simulink model "sim_inverter_MA"  (R2022a)
settings: Solver=FixedStepDiscrete  StartTime=0.0  StopTime=5  FixedStep=Ts  RelTol=1e-3
PreLoadFcn:
  | sim_params;
InitFcn:
  | sim_params;
values from neighbouring files (symbols this model uses):
  capacitor_C = 0.00033    [sim_datadict.sldd]
  capacitor_R = 0.03    [sim_datadict.sldd]
  freq_ref = 60.0    [sim_datadict.sldd]
  fsw = 10000    [run_simulation.m]    (also in sim_params.m)
  I_ref = 6.5    [sim_datadict.sldd]
  Ki_i = 36.06    [sim_params.m]
  Ki_vd = Ki    (= 341.85)    [sim_params.m]
  Ki_vq = Ki    (= 341.85)    [sim_params.m]
  Kp_i = 0.0405    [sim_params.m]
  Kp_vd = Kp    (= 3.68799083448)    [sim_params.m]
  Kp_vq = Kp    (= 3.68799083448)    [sim_params.m]
  source_L = {0, 0.3e-3, 0.6e-3, 1e-3, 1.8e-3, 3.5e-3, 5e-3, 8e-3, 15e-3, 25e-3, 165e-3}    [load_sim_space.m]    (also in run_inverterSims.m = {0, 0.3e-3, 0.6e-3, 1e-3, 1.8e-3, 3.5e-3, 5e-3, 8e-3, 15e-3,; sim_datadict.sldd = 0.001)
  source_R = {0, 0.1, 0.2, 0.3, 0.5, 1, 1.5, 2.5, 5, 8, 12.5}    [load_sim_space.m]    (also in run_inverterSims.m = {0, 0.1, 0.2, 0.3, 0.5, 1, 1.5, 2.5, 5, 8}; sim_datadict.sldd = 0.1)
  Ts = 1e-6    (= 1e-06)    [run_simulation.m]    (also in sim_params.m)
  Vref = 380    [load_control_params.m]    (also in sim_params.m)
libraries: slpidlib x3, spsRMSLib x3, spsThreePhaseVIMeasurementLib x2, spsAsynchronousMachineSIUnitsLib x1, spsAlphaBetaZerotoabcLib x1, spsAlphaBetaZerotodq0Lib x1, eeAsmScalarControl x1, eeGeneralControl x1, eePwmGeneratorTwoLevel x1, spsabctoAlphaBetaZeroLib x1, spsdq0toAlphaBetaZeroLib x1, spsThreePhaseSourceLib x1
settings Model: DataDictionary=sim_datadict.sldd  ARTEMISmethode_block_infos=$$__separator__$$  SimulationMode=accelerator  Creator=thale  LastModifiedBy=thale
settings DataIOCC: LimitDataPoints=on  MaxDataPoints=1/Ts  SaveFormat=Array  SaveOutput=off  DSMLogging=off  SaveTime=off  ReturnWorkspaceOutputs=off  TimeSaveName=time  LoggingIntervals=[0, inf]

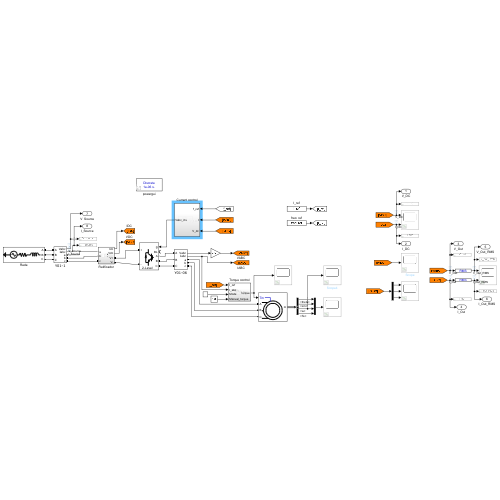
[thumbnail: Simulink's stored preview of the top-level diagram]
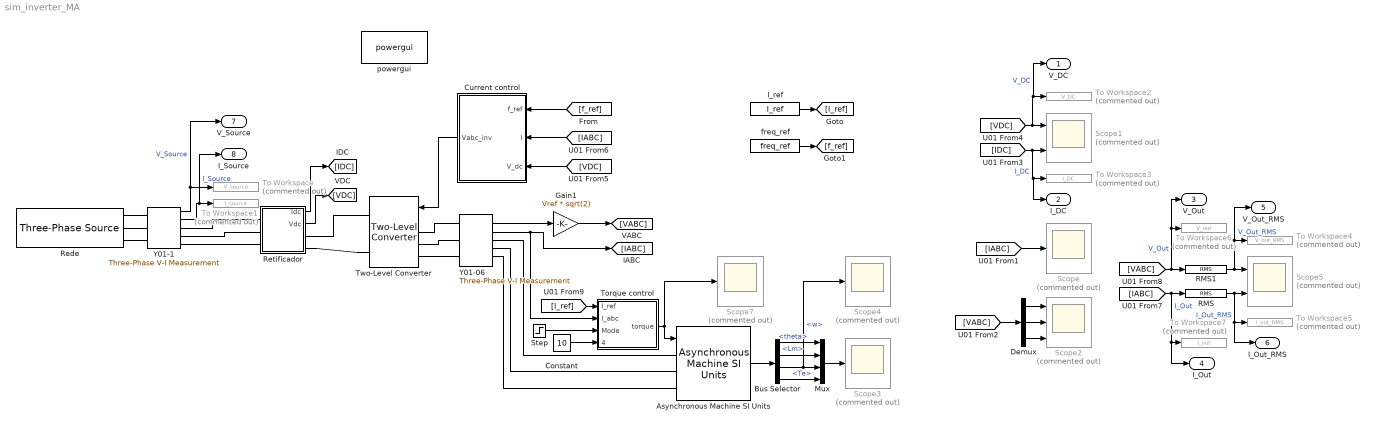
== system sim_inverter_MA ==
  Asynchronous Machine SI Units : spsAsynchronousMachineSIUnitsLib/Asynchronous Machine SI Units  RotorType=Squirrel-cage  PresetModel=No  MechanicalLoad=Torque Tm  ShowDetailedParameters=on  ReferenceFrame=Rotor  Units=SI  MeasurementBus=on  NominalParameters=[3000 380 60]  VoltageRatio=1  Stator=[0.6837 0.004152]  Rotor=[0.451 0.004152]  Cage1=[0.4155 0.002066]  Cage2=[0.4168 0.0003495]  Lm=0.1486  Mechanical=[0.0120 0.008141 2]  PolePairs=2  InitialConditions=[0 0 0 0 0 0 0 0]  SimulateSaturation=off  Saturation=[14.03593122, 27.81365428, 53.79336849, 72.68890987, 97.98006896, 148.6815601, 215.7428561, 302.9841135, 428.7778367 ; 230, 322, 414, 460, 506, 552, 598, 644, 690]  LoadFlowParameters=1492000  TsPowergui=0  TsBlock=-1  IterativeModel=Trapezoidal non iterative  IterativeDiscreteModel=Trapezoidal non iterative  Pmec=1.492e+006
  Bus Selector : BusSelector  OutputSignals=theta,Lm,w,Te
  Constant : Constant  Value=10
  Current control : Subsystem
  Demux : Demux  Outputs=3
  Gain1 : Gain  Gain=Vref * sqrt(2)
  I_ref : Constant  Value=I_ref
  Mux : Mux
  RMS : spsRMSLib/RMS  TrueRMS=off  Freq=freq_ref  RMSInit=0  Ts=Ts
  RMS1 : spsRMSLib/RMS  TrueRMS=off  Freq=freq_ref  RMSInit=0  Ts=Ts
  Rede : spsThreePhaseSourceLib/Three-Phase Source  InternalConnection=Yg  VoltagePhases=off  Voltage=Vref  PhaseAngle=0  Voltage_phases=[25e3 25e3 25e3]/sqrt(3)  PhaseAngles_phases=[0 -120 +120]  Frequency=60  NonIdealSource=on  SpecifyImpedance=off  Resistance=source_R  Inductance=source_L  ShortCircuitLevel=100e6  BaseVoltage=Vref  XRratio=7  BusType=swing  Pref=10e3  Qref=0  Prefabc=[10e3, 10e3, 10e3]  Qrefabc=[0, 0, 0]  Qmin=-inf  Qmax=inf
  Retificador : Subsystem
  Scope{,3..4,7} (4 alike) : Scope  Commented=on
  Scope1 : Scope  Commented=on  NumInputPorts=2
  Scope2 : Scope  Commented=on  NumInputPorts=3
  Scope5 : Scope  Commented=on  NumInputPorts=2
  Step : Step  Time=0.5  SampleTime=0
  To Workspace : ToWorkspace  Commented=on  VariableName=V_source  SampleTime=-1
      settings: MaxDataPoints=1/Ts  Save2DSignal=2-D array (concatenate along first dimension)
  To Workspace1 : ToWorkspace  Commented=on  VariableName=I_source  SampleTime=-1
      settings: Save2DSignal=2-D array (concatenate along first dimension)
  To Workspace2 : ToWorkspace  Commented=on  VariableName=V_DC  SampleTime=-1
      settings: MaxDataPoints=1/Ts  Save2DSignal=2-D array (concatenate along first dimension)
  To Workspace3 : ToWorkspace  Commented=on  VariableName=I_DC  SampleTime=-1
      settings: MaxDataPoints=1/Ts  Save2DSignal=2-D array (concatenate along first dimension)
  To Workspace4 : ToWorkspace  Commented=on  VariableName=V_out_RMS  SampleTime=-1
      settings: MaxDataPoints=1/Ts  Save2DSignal=2-D array (concatenate along first dimension)
  To Workspace5 : ToWorkspace  Commented=on  VariableName=I_out_RMS  SampleTime=-1
      settings: Save2DSignal=2-D array (concatenate along first dimension)
  To Workspace6 : ToWorkspace  Commented=on  VariableName=V_out  SampleTime=-1
      settings: MaxDataPoints=1/Ts  Save2DSignal=2-D array (concatenate along first dimension)
  To Workspace7 : ToWorkspace  Commented=on  VariableName=I_out  SampleTime=-1
      settings: MaxDataPoints=1/Ts  Save2DSignal=2-D array (concatenate along first dimension)
  Torque control : Subsystem
  Two-Level Converter : spsTwoLevelConverterLib/Two-Level Converter  ModelType=Switching devices  Ron=1e-3  Rs=1e6  Cs=inf  Vforward=[0,0]  Ron_Diode=1e-3  Rs_Diode=1e6  Cs_Diode=inf  Vf_Diode=1e-3  Rs_CurrentSource=inf  Ron_ACsource=1e-3
      settings: SourceProductBaseCode=PS
  Y01-06 : spsThreePhaseVIMeasurementLib/Three-Phase V-I Measurement  VoltageMeasurement=phase-to-ground  SetLabelV=off  LabelV=Vabc  Vpu=on  VpuLL=off  CurrentMeasurement=yes  SetLabelI=off  LabelI=Iabc  Ipu=off  Pbase=100e6  Vbase=Vref  OutputType=Complex  PhasorSimulation=off  PSBequivalent=0
  Y01-1 : spsThreePhaseVIMeasurementLib/Three-Phase V-I Measurement  VoltageMeasurement=phase-to-ground  SetLabelV=off  LabelV=Vabc  Vpu=off  VpuLL=off  CurrentMeasurement=yes  SetLabelI=off  LabelI=Iabc  Ipu=off  Pbase=100e6  Vbase=Vref  OutputType=Complex  PhasorSimulation=off  PSBequivalent=0
  freq_ref : Constant  Value=freq_ref
  powergui : spspowerguiLib/powergui  Priority=1  SimulationMode=Discrete  SampleTime=Ts  frequency=60  Iterations=50  frequencyindice=0  Pbase=100e6  ErrMax=1e-4  UnitsV=kV  UnitsW=MW  buscounter=0  FunctionMessages=off  echomessages=off  EnableUseOfTLC=off  CurrentSourceSwitches=off  DisableSnubberDevices=off  DisableRonSwitches=off  DisableVfSwitches=off  DisplayEquations=off  AutomaticDiscreteSolvers=off  SolverType=Tustin/Backward Euler (TBE)  Interpol=off  ExternalGateDelay=off  methode=off  Ts=100  x0status=blocks  SPID=on  SwTol=0  HookPort=off  NonlinearTolerance=1e-4  nMaxIteration=100  ContinueOnMaxIteration=off  RestoreLinks=warning  ResistiveCurrentMeasurement=off  Frange=[0:2:500]  Ylog=off  Xlog=on  ShowGrid=off  save=off  variable=ZData  structure=0  ZoomFFT=off  StartTime=0.0  cycles=1  DisplayStyle=1  fundamental=60  FreqAxis=off  MaxFrequency=1000  frequencyindicesteady=1  RmsSteady=1  display=off
  V_DC : Outport
  I_DC : Outport  Port=2
  V_Out : Outport  Port=3
  I_Out : Outport  Port=4
  V_Out_RMS : Outport  Port=5
  I_Out_RMS : Outport  Port=6
  V_Source : Outport  Port=7
  I_Source : Outport  Port=8
  wires:
  [IABC] -> Scope/1
  Y01-06/2 -> Torque control/2(I_abc), [IABC]
  [IDC] -> I_DC/1, To Workspace3/1, Scope1/2  "I_DC"
  [VDC] -> V_DC/1, To Workspace2/1, Scope1/1  "V_DC"
  Demux/1 -> Scope2/1
  Demux/2 -> Scope2/2
  Demux/3 -> Scope2/3
  Asynchronous Machine SI Units/1 -> Bus Selector/1
  Bus Selector/4 -> Mux/4  "<Te>"
  Bus Selector/2 -> Mux/2  "<Lm>"
  Bus Selector/3 -> Scope4/1, Mux/3  "<w>"
  Mux/1 -> Scope3/1
  Bus Selector/1 -> Mux/1  "<theta>"
  Y01-06/1 -> Gain1/1
  Gain1/1 -> [VABC]
  Current control/1(Vabc_inv) -> Two-Level Converter/1
  [VABC] -> Demux/1
  Retificador/1(Idc) -> [IDC]
  Retificador/2(Vdc) -> [VDC]
  [VDC] -> Current control/3(V_dc)
  [f_ref] -> Current control/1(f_ref)
  [IABC] -> Current control/2(I)
  RMS1/1 -> V_Out_RMS/1, To Workspace4/1, Scope5/1  "V_Out_RMS"
  RMS/1 -> I_Out_RMS/1, To Workspace5/1, Scope5/2  "I_Out_RMS"
  [VABC] -> V_Out/1, To Workspace6/1, RMS1/1  "V_Out"
  [IABC] -> I_Out/1, To Workspace7/1, RMS/1  "I_Out"
  I_ref/1 -> [I_ref]
  freq_ref/1 -> [f_ref]
  [I_ref] -> Torque control/1(I_ref)
  Step/1 -> Torque control/3(Mode)
  Constant/1 -> Torque control/4(Manual_torque)
  Y01-1/1 -> V_Source/1, To Workspace/1  "V_Source"
  Y01-1/2 -> I_Source/1, To Workspace1/1  "I_Source"
  Torque control/1(torque) -> Asynchronous Machine SI Units/1, Scope7/1
  connections:
  Asynchronous Machine SI Units/LConn3 -- Y01-06/RConn3
  Asynchronous Machine SI Units/LConn1 -- Y01-06/RConn1
  Asynchronous Machine SI Units/LConn2 -- Y01-06/RConn2
  Retificador/RConn1 -- Two-Level Converter/RConn1
  Retificador/RConn2 -- Two-Level Converter/RConn2
  Y01-1/LConn1 -- Rede/RConn1
  Y01-1/LConn2 -- Rede/RConn2
  Y01-1/LConn3 -- Rede/RConn3
  Y01-1/RConn1 -- Retificador/LConn1
  Retificador/LConn2 -- Y01-1/RConn2
  Y01-1/RConn3 -- Retificador/LConn3
  Y01-06/LConn1 -- Two-Level Converter/LConn1
  Y01-06/LConn2 -- Two-Level Converter/LConn2
  Y01-06/LConn3 -- Two-Level Converter/LConn3

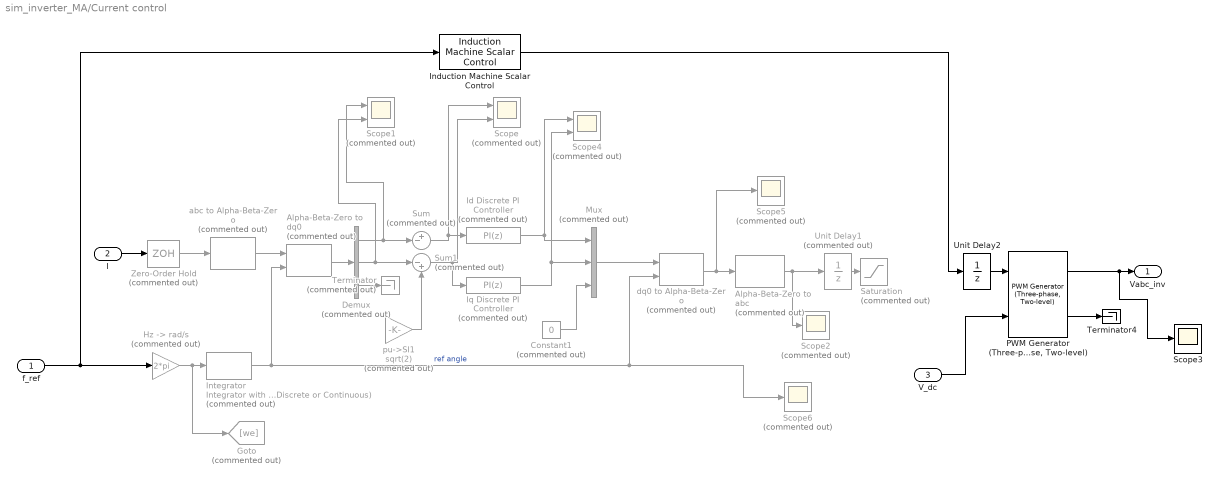
== system sim_inverter_MA/Current control ==
  f_ref : Inport
  I : Inport  Port=2
  V_dc : Inport  Port=3
  Alpha-Beta-Zero to abc : spsAlphaBetaZerotoabcLib/Alpha-Beta-Zero to abc  Commented=on
      settings: SourceProductBaseCode=PS
  Alpha-Beta-Zero to dq0 : spsAlphaBetaZerotodq0Lib/Alpha-Beta-Zero to dq0  Commented=on  Alignment=90 degrees behind phase A axis
      settings: SourceProductBaseCode=PS
  Constant1 : Constant  Commented=on  Value=0
  Demux : Demux  Commented=on  Outputs=3
  Goto : Goto  Commented=on  GotoTag=we
  "Hz -> rad/s" : Gain  Commented=on  Gain=2*pi
  Id Discrete PI Controller : slpidlib/PID Controller  Commented=on  Controller=PI  Form=Parallel  TimeDomain=Discrete-time  UseExternalTs=off  SampleTime=1/fsw  IntegratorMethod=Forward Euler  FilterMethod=Forward Euler  ControllerParametersSource=internal  P=Kp_vd  I=Ki_vd  UseKiTs=off  D=0  N=100  UseFilter=on  TunerSelectOption=Transfer Function Based (PID Tuner App)  InitialConditionSource=internal  InitialConditionForIntegrator=0.5  InitialConditionForFilter=0  DifferentiatorICPrevScaledInput=0  ExternalReset=none  TrackingMode=off  Kt=1  LimitOutput=off  SatLimitsSource=internal  UpperSaturationLimit=inf  LowerSaturationLimit=-1000  LinearizeAsGain=on  AntiWindupMode=none  Kb=1  POutMin=[]  POutMax=[]  IOutMin=[]  IOutMax=[]  DOutMin=[]  DOutMax=[]  NOutMin=[]  NOutMax=[]  SumOutMin=[]  SumOutMax=[]  SaturationOutMin=[]  SaturationOutMax=[]  PParamMin=[]  PParamMax=[]  IParamMin=[]  IParamMax=[]  DParamMin=[]  DParamMax=[]  NParamMin=[]  NParamMax=[]  KbParamMin=[]  KbParamMax=[]  KtParamMin=[]  KtParamMax=[]  KbOutMin=[]  KbOutMax=[]  KtOutMin=[]  KtOutMax=[]  IntegratorOutMin=[]  IntegratorOutMax=[]  FilterOutMin=[]  FilterOutMax=[]  SumI1OutMin=[]  SumI1OutMax=[]  SumI2OutMin=[]  SumI2OutMax=[]  SumI3OutMin=[]  SumI3OutMax=[]  SumI4OutMin=[]  SumI4OutMax=[]  SumDOutMin=[]  SumDOutMax=[]  DifferentiatorOutMin=[]  DifferentiatorOutMax=[]  FilterDiffOutCoefMin=[]  FilterDiffOutCoefMax=[]  ReciprocalOutMin=[]  ReciprocalOutMax=[]  SumDenOutMin=[]  SumDenOutMax=[]  SumNumOutMin=[]  SumNumOutMax=[]  DivideOutMin=[]  DivideOutMax=[]  UdiffTsProdOutMin=[]  UdiffTsProdOutMax=[]  NTsProdOutMin=[]  NTsProdOutMax=[]  UintegralTsProdOutMin=[]  UintegralTsProdOutMax=[]  UngainTsProdOutMin=[]  UngainTsProdOutMax=[]  ClampingZeroOutDataTypeStr=Inherit: Inherit via back propagation  ClampingZeroOutMin=[]  ClampingZeroOutMax=[]  FilterDenConstantOutDataTypeStr=Inherit: Inherit via back propagation  FilterDenConstantOutMin=[]  FilterDenConstantOutMax=[]  PCopyOutDataTypeStr=Inherit: Inherit via back propagation  PCopyOutMin=[]  PCopyOutMax=[]  NCopyOutDataTypeStr=Inherit: Inherit via back propagation  NCopyOutMin=[]  NCopyOutMax=[]  IntegratorContinuousStateAttributes=''  IntegratorStateMustResolveToSignalObject=off  IntegratorRTWStateStorageClass=Auto  FilterContinuousStateAttributes=''  FilterStateMustResolveToSignalObject=off  FilterRTWStateStorageClass=Auto  ParallelPVariant=InternalParameters  IdealPVariant=Disabled  IVariant=InternalParameters  DVariant=Disabled  IntegratorVariant=Discrete  SatVariant=Disabled  AWVariant=Passthrough  PCopyVariant=Disabled  TRVariant=Disabled  FdbkBlocksVariant=Forward  IdealPFdbkVariant=Disabled  SatFdbkVariant=Disabled  DerivativeFilterVariant=Disabled  NVariant=Disabled  NCopyVariant=Disabled_SignalSpec  FilterICVariant=Disabled  IntegratorICVariant=InternalICs  ExternalResetVariant=Disabled  TRSumVariant=Passthrough  SumFdbkVariant=Disabled  SumVariant=Sum_PI  TsampFilterVariant=InternalTs  TsampNgainVariant=Passthrough  TsampIntegralVariant=Passthrough  ExternalSaturationOutDataTypeStr=Inherit: Same as second input  aMode=0
  Induction Machine Scalar Control : eeAsmScalarControl/Induction Machine Scalar Control  fn=60  Vn=220  Vmin=20  Ts=-1
      settings: SourceProductBaseCode=PS
  Integrator : eeGeneralControl/Integrator with Wrapped State (Discrete or Continuous)  Commented=on  LabelModeActiveChoice=Discrete  WrappedStateUpperValue=2*pi  WrappedStateLowerValue=0  x0=0  Ts=1/fsw
      settings: SourceProductBaseCode=PS
  Iq Discrete PI Controller : slpidlib/PID Controller  Commented=on  Controller=PI  Form=Parallel  TimeDomain=Discrete-time  UseExternalTs=off  SampleTime=1/fsw  IntegratorMethod=Forward Euler  FilterMethod=Forward Euler  ControllerParametersSource=internal  P=Kp_vq  I=Ki_vq  UseKiTs=off  D=0  N=100  UseFilter=on  TunerSelectOption=Transfer Function Based (PID Tuner App)  InitialConditionSource=internal  InitialConditionForIntegrator=1  InitialConditionForFilter=0  DifferentiatorICPrevScaledInput=0  ExternalReset=none  TrackingMode=off  Kt=1  LimitOutput=off  SatLimitsSource=internal  UpperSaturationLimit=inf  LowerSaturationLimit=-100  LinearizeAsGain=on  AntiWindupMode=none  Kb=1  POutMin=[]  POutMax=[]  IOutMin=[]  IOutMax=[]  DOutMin=[]  DOutMax=[]  NOutMin=[]  NOutMax=[]  SumOutMin=[]  SumOutMax=[]  SaturationOutMin=[]  SaturationOutMax=[]  PParamMin=[]  PParamMax=[]  IParamMin=[]  IParamMax=[]  DParamMin=[]  DParamMax=[]  NParamMin=[]  NParamMax=[]  KbParamMin=[]  KbParamMax=[]  KtParamMin=[]  KtParamMax=[]  KbOutMin=[]  KbOutMax=[]  KtOutMin=[]  KtOutMax=[]  IntegratorOutMin=[]  IntegratorOutMax=[]  FilterOutMin=[]  FilterOutMax=[]  SumI1OutMin=[]  SumI1OutMax=[]  SumI2OutMin=[]  SumI2OutMax=[]  SumI3OutMin=[]  SumI3OutMax=[]  SumI4OutMin=[]  SumI4OutMax=[]  SumDOutMin=[]  SumDOutMax=[]  DifferentiatorOutMin=[]  DifferentiatorOutMax=[]  FilterDiffOutCoefMin=[]  FilterDiffOutCoefMax=[]  ReciprocalOutMin=[]  ReciprocalOutMax=[]  SumDenOutMin=[]  SumDenOutMax=[]  SumNumOutMin=[]  SumNumOutMax=[]  DivideOutMin=[]  DivideOutMax=[]  UdiffTsProdOutMin=[]  UdiffTsProdOutMax=[]  NTsProdOutMin=[]  NTsProdOutMax=[]  UintegralTsProdOutMin=[]  UintegralTsProdOutMax=[]  UngainTsProdOutMin=[]  UngainTsProdOutMax=[]  ClampingZeroOutDataTypeStr=Inherit: Inherit via back propagation  ClampingZeroOutMin=[]  ClampingZeroOutMax=[]  FilterDenConstantOutDataTypeStr=Inherit: Inherit via back propagation  FilterDenConstantOutMin=[]  FilterDenConstantOutMax=[]  PCopyOutDataTypeStr=Inherit: Inherit via back propagation  PCopyOutMin=[]  PCopyOutMax=[]  NCopyOutDataTypeStr=Inherit: Inherit via back propagation  NCopyOutMin=[]  NCopyOutMax=[]  IntegratorContinuousStateAttributes=''  IntegratorStateMustResolveToSignalObject=off  IntegratorRTWStateStorageClass=Auto  FilterContinuousStateAttributes=''  FilterStateMustResolveToSignalObject=off  FilterRTWStateStorageClass=Auto  ParallelPVariant=InternalParameters  IdealPVariant=Disabled  IVariant=InternalParameters  DVariant=Disabled  IntegratorVariant=Discrete  SatVariant=Disabled  AWVariant=Passthrough  PCopyVariant=Disabled  TRVariant=Disabled  FdbkBlocksVariant=Forward  IdealPFdbkVariant=Disabled  SatFdbkVariant=Disabled  DerivativeFilterVariant=Disabled  NVariant=Disabled  NCopyVariant=Disabled_SignalSpec  FilterICVariant=Disabled  IntegratorICVariant=InternalICs  ExternalResetVariant=Disabled  TRSumVariant=Passthrough  SumFdbkVariant=Disabled  SumVariant=Sum_PI  TsampFilterVariant=InternalTs  TsampNgainVariant=Passthrough  TsampIntegralVariant=Passthrough  ExternalSaturationOutDataTypeStr=Inherit: Same as second input  aMode=0
  Mux : Mux  Commented=on  Inputs=3
  "PWM Generator (Three-phase, Two-level)" : eePwmGeneratorTwoLevel/PWM Generator (Three-phase, Two-level)  PWMMode=Continuous PWM (CPWM)  CPWMMode=SPWM: sinusoidal PWM  DPWMMode=60 DPWM: 60 degree discontinuous PWM  fsw=fsw  Ts=Ts
      settings: SourceProductBaseCode=PS
  Saturation : Saturate  Commented=on
  Scope : Scope  Commented=on  NumInputPorts=2
  Scope1 : Scope  Commented=on  NumInputPorts=2
  Scope2 : Scope  Commented=on
  Scope3 : Scope
  Scope4 : Scope  Commented=on  NumInputPorts=2
  Scope5 : Scope  Commented=on
  Scope6 : Scope  Commented=on
  Sum : Sum  Commented=on  Inputs=+-|
  Sum1 : Sum  Commented=on  Inputs=|-+
  Terminator : Terminator  Commented=on
  Terminator4 : Terminator
  Unit Delay1 : UnitDelay  Commented=on  SampleTime=1/fsw  HasFrameUpgradeWarning=on
  Unit Delay2 : UnitDelay  SampleTime=1/fsw  HasFrameUpgradeWarning=on
  Zero-Order Hold : ZeroOrderHold  Commented=on  SampleTime=1/fsw
  abc to Alpha-Beta-Zero : spsabctoAlphaBetaZeroLib/abc to Alpha-Beta-Zero  Commented=on
      settings: SourceProductBaseCode=PS
  dq0 to Alpha-Beta-Zero : spsdq0toAlphaBetaZeroLib/dq0 to Alpha-Beta-Zero  Commented=on  Alignment=90 degrees behind phase A axis
      settings: SourceProductBaseCode=PS
  pu->SI1 : Gain  Commented=on  Gain=sqrt(2)
  Vabc_inv : Outport
  wires:
  abc to Alpha-Beta-Zero/1 -> Alpha-Beta-Zero to dq0/1
  I/1 -> Zero-Order Hold/1
  Alpha-Beta-Zero to dq0/1 -> Demux/1
  Demux/3 -> Terminator/1
  Sum/1 -> Scope/1, Id Discrete PI Controller/1
  Sum1/1 -> Scope/2, Iq Discrete PI Controller/1
  Constant1/1 -> Mux/3
  Mux/1 -> dq0 to Alpha-Beta-Zero/1
  Integrator/1 -> Alpha-Beta-Zero to dq0/2, Scope6/1, dq0 to Alpha-Beta-Zero/2  "ref angle"
  "PWM Generator (Three-phase, Two-level)"/2 -> Terminator4/1
  ? -> pu->SI1/1
  pu->SI1/1 -> Sum1/2
  dq0 to Alpha-Beta-Zero/1 -> Alpha-Beta-Zero to abc/1, Scope5/1
  V_dc/1 -> "PWM Generator (Three-phase, Two-level)"/2
  Zero-Order Hold/1 -> abc to Alpha-Beta-Zero/1
  Alpha-Beta-Zero to abc/1 -> Scope2/1, Unit Delay1/1
  "PWM Generator (Three-phase, Two-level)"/1 -> Scope3/1, Vabc_inv/1
  Demux/2 -> Sum1/1, Scope1/2
  Demux/1 -> Scope1/1, Sum/2
  Iq Discrete PI Controller/1 -> Mux/2, Scope4/2
  Id Discrete PI Controller/1 -> Mux/1, Scope4/1
  "Hz -> rad/s"/1 -> Goto/1, Integrator/1
  Unit Delay1/1 -> Saturation/1
  Induction Machine Scalar Control/1 -> Unit Delay2/1
  Unit Delay2/1 -> "PWM Generator (Three-phase, Two-level)"/1
  f_ref/1 -> Induction Machine Scalar Control/1, "Hz -> rad/s"/1

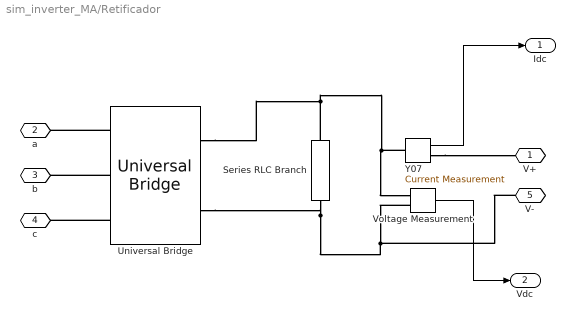
== system sim_inverter_MA/Retificador ==
  Series RLC Branch : spsSeriesRLCBranchLib/Series RLC Branch  LConnTagsString=__new0  RConnTagsString=__new0  BranchType=RC  Resistance=capacitor_R  Inductance=1e-3  SetiL0=off  InitialCurrent=0  Capacitance=capacitor_C  Setx0=off  InitialVoltage=0  Measurements=None
  Universal Bridge : spsUniversalBridgeLib/Universal Bridge  Arms=3  SnubberResistance=1e5  SnubberCapacitance=inf  Device=Diodes  Ron=1e-3  Lon=0  ForwardVoltages="[  0  0  ]"  ForwardVoltage=0.8  GTOparameters=[ 10e-6 , 20e-6 ]  IGBTparameters=[ 1e-6 , 2e-6 ]  Measurements=None  Measurements_2=None  converterType=Rectifier
  Voltage Measurement : spsVoltageMeasurementLib/Voltage Measurement  PhasorSimulation=off  OutputType=Complex  PSBequivalent=0
  Y07 : spsCurrentMeasurementLib/Current Measurement  PhasorSimulation=off  OutputType=Complex  PSBequivalent=0
  V+ : PMIOPort  Side=Right
  a : PMIOPort  Port=2  Side=Left
  b : PMIOPort  Port=3  Side=Left
  c : PMIOPort  Port=4  Side=Left
  V- : PMIOPort  Port=5  Side=Right
  Idc : Outport
  Vdc : Outport  Port=2
  wires:
  Y07/1 -> Idc/1
  Voltage Measurement/1 -> Vdc/1
  connections:
  Series RLC Branch/RConn1 -- Y07/LConn1 -- Voltage Measurement/LConn1 -- Universal Bridge/RConn1
  Series RLC Branch/LConn1 -- V-/RConn1 -- Voltage Measurement/LConn2 -- Universal Bridge/RConn2
  Y07/RConn1 -- V+/RConn1
  Universal Bridge/LConn3 -- c/RConn1
  Universal Bridge/LConn2 -- b/RConn1
  Universal Bridge/LConn1 -- a/RConn1

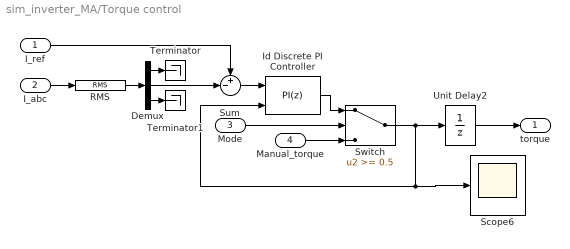
== system sim_inverter_MA/Torque control ==
  I_ref : Inport
  I_abc : Inport  Port=2
  Mode : Inport  Port=3
  Manual_torque : Inport  Port=4
  Demux : Demux  Outputs=3
  Id Discrete PI Controller : slpidlib/PID Controller  Controller=PI  Form=Parallel  TimeDomain=Discrete-time  UseExternalTs=off  SampleTime=Ts  IntegratorMethod=Forward Euler  FilterMethod=Forward Euler  ControllerParametersSource=internal  P=Kp_i  I=Ki_i  UseKiTs=off  D=0  N=100  UseFilter=on  TunerSelectOption=Transfer Function Based (PID Tuner App)  InitialConditionSource=internal  InitialConditionForIntegrator=0.5  InitialConditionForFilter=0  DifferentiatorICPrevScaledInput=0  ExternalReset=none  TrackingMode=on  Kt=1  LimitOutput=on  SatLimitsSource=internal  UpperSaturationLimit=inf  LowerSaturationLimit=0  LinearizeAsGain=off  AntiWindupMode=clamping  Kb=1  POutMin=[]  POutMax=[]  IOutMin=[]  IOutMax=[]  DOutMin=[]  DOutMax=[]  NOutMin=[]  NOutMax=[]  SumOutMin=[]  SumOutMax=[]  SaturationOutMin=[]  SaturationOutMax=[]  PParamMin=[]  PParamMax=[]  IParamMin=[]  IParamMax=[]  DParamMin=[]  DParamMax=[]  NParamMin=[]  NParamMax=[]  KbParamMin=[]  KbParamMax=[]  KtParamMin=[]  KtParamMax=[]  KbOutMin=[]  KbOutMax=[]  KtOutMin=[]  KtOutMax=[]  IntegratorOutMin=[]  IntegratorOutMax=[]  FilterOutMin=[]  FilterOutMax=[]  SumI1OutMin=[]  SumI1OutMax=[]  SumI2OutMin=[]  SumI2OutMax=[]  SumI3OutMin=[]  SumI3OutMax=[]  SumI4OutMin=[]  SumI4OutMax=[]  SumDOutMin=[]  SumDOutMax=[]  DifferentiatorOutMin=[]  DifferentiatorOutMax=[]  FilterDiffOutCoefMin=[]  FilterDiffOutCoefMax=[]  ReciprocalOutMin=[]  ReciprocalOutMax=[]  SumDenOutMin=[]  SumDenOutMax=[]  SumNumOutMin=[]  SumNumOutMax=[]  DivideOutMin=[]  DivideOutMax=[]  UdiffTsProdOutMin=[]  UdiffTsProdOutMax=[]  NTsProdOutMin=[]  NTsProdOutMax=[]  UintegralTsProdOutMin=[]  UintegralTsProdOutMax=[]  UngainTsProdOutMin=[]  UngainTsProdOutMax=[]  ClampingZeroOutDataTypeStr=Inherit: Inherit via back propagation  ClampingZeroOutMin=[]  ClampingZeroOutMax=[]  FilterDenConstantOutDataTypeStr=Inherit: Inherit via back propagation  FilterDenConstantOutMin=[]  FilterDenConstantOutMax=[]  PCopyOutDataTypeStr=Inherit: Inherit via back propagation  PCopyOutMin=[]  PCopyOutMax=[]  NCopyOutDataTypeStr=Inherit: Inherit via back propagation  NCopyOutMin=[]  NCopyOutMax=[]  IntegratorContinuousStateAttributes=''  IntegratorStateMustResolveToSignalObject=off  IntegratorRTWStateStorageClass=Auto  FilterContinuousStateAttributes=''  FilterStateMustResolveToSignalObject=off  FilterRTWStateStorageClass=Auto  ParallelPVariant=InternalParameters  IdealPVariant=Disabled  IVariant=InternalParameters  DVariant=Disabled  IntegratorVariant=Discrete  SatVariant=Enabled  AWVariant=DiscClampingParallel  PCopyVariant=Disabled  TRVariant=Enabled  FdbkBlocksVariant=Forward  IdealPFdbkVariant=Disabled  SatFdbkVariant=Disabled  DerivativeFilterVariant=Disabled  NVariant=Disabled  NCopyVariant=Disabled_SignalSpec  FilterICVariant=Disabled  IntegratorICVariant=InternalICs  ExternalResetVariant=Disabled  TRSumVariant=TrackingMode  SumFdbkVariant=Disabled  SumVariant=Sum_PI  TsampFilterVariant=InternalTs  TsampNgainVariant=Passthrough  TsampIntegralVariant=Passthrough  ExternalSaturationOutDataTypeStr=Inherit: Same as second input  aMode=0
  RMS : spsRMSLib/RMS  TrueRMS=off  Freq=freq_ref  RMSInit=0  Ts=Ts
  Scope6 : Scope
  Sum : Sum  Inputs=+-|
  Switch : Switch  Threshold=0.5  SaturateOnIntegerOverflow=off  InputSameDT=off
  Terminator : Terminator
  Terminator1 : Terminator
  Unit Delay2 : UnitDelay  SampleTime=-1  HasFrameUpgradeWarning=on
  torque : Outport
  wires:
  Unit Delay2/1 -> torque/1
  Sum/1 -> Id Discrete PI Controller/1
  I_abc/1 -> RMS/1
  I_ref/1 -> Sum/1
  RMS/1 -> Demux/1
  Demux/2 -> Sum/2
  Switch/1 -> Id Discrete PI Controller/2, Scope6/1, Unit Delay2/1
  Id Discrete PI Controller/1 -> Switch/1
  Mode/1 -> Switch/2
  Manual_torque/1 -> Switch/3
  Demux/1 -> Terminator/1
  Demux/3 -> Terminator1/1
